simulink model "practica3sim"  (R2015a)
settings: Solver=ode45  StartTime=0.0  StopTime=20  RelTol=1e-3
settings Model: Creator=Sala6  LastModifiedBy=Sala6

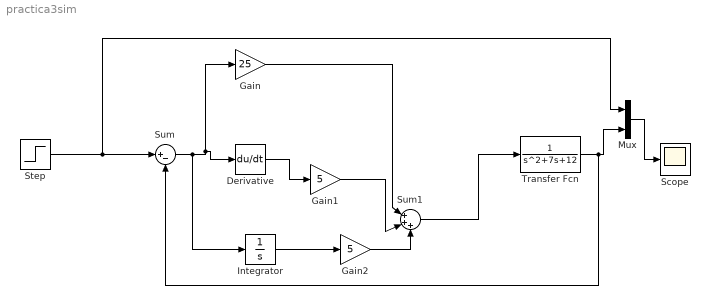
== system practica3sim ==
  Derivative : Derivative
  Gain : Gain  Gain=25
  Gain1 : Gain  Gain=5
  Gain2 : Gain  Gain=5
  Integrator : Integrator
  Mux : Mux  Inputs=2
  Scope : Scope
  Step : Step  After=5  SampleTime=0
  Sum : Sum  Inputs=|+-
  Sum1 : Sum  Inputs=|+++
  Transfer Fcn : TransferFcn  Denominator=[1 7 12]
  wires:
  Mux/1 -> Scope/1
  Transfer Fcn/1 -> Sum/2, Mux/2
  Step/1 -> Mux/1, Sum/1
  Sum/1 -> Integrator/1, Derivative/1, Gain/1
  Derivative/1 -> Gain1/1
  Integrator/1 -> Gain2/1
  Gain/1 -> Sum1/1
  Gain1/1 -> Sum1/2
  Sum1/1 -> Transfer Fcn/1
  Gain2/1 -> Sum1/3
